simulink model "mass"  (R2025b)
settings: Solver=VariableStepAuto  StartTime=0.0  StopTime=10.0  RelTol=1e-3
PostLoadFcn:
  | rigid_body = importrobot('urdf\mass\urdf\mass.urdf');
  | rigid_body.DataFormat = 'column';
  | rigid_body.Gravity = [0 -9.81 0];
  | robot = get_robot_chain(rigid_body, 'mass','base_link');
  | robot.gravity = [0 -9.81 0];
libraries: aerolibanimutils x1
settings Model: Creator=Junch  LastModifiedBy=Junch

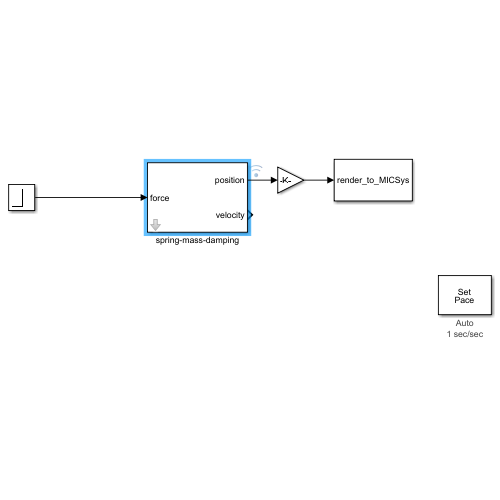
[thumbnail: Simulink's stored preview of the top-level diagram]
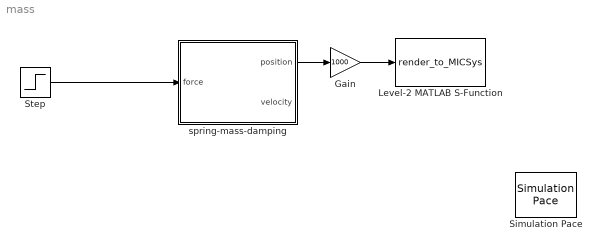
== system mass ==
  Gain : Gain  Gain=1000
  Level-2 MATLAB S-Function : M-S-Function  FunctionName=render_to_MICSys
  Simulation Pace : aerolibanimutils/Simulation Pace  SimulationPace=1  SleepMode=Auto  OutputPaceError=off  SampleTime=1/30
  Step : Step  SampleTime=0
  spring-mass-damping : Subsystem  mask{robot=robot, x0=0, Kd=1, Kp=5}
      mask prompts: x0 "intial position"; Kd "Kd (damping)"; Kp "Kp (spring)"
      mask DialogControl ParameterGroupVar Prompt: 参数
      mask Display:
      | port_label('output', 1, 'position');
      | port_label('output', 2, 'velocity');
      | port_label('input', 1, 'force');
  wires:
  Step/1 -> spring-mass-damping/1(force)
  spring-mass-damping/1(position) -> Gain/1
  Gain/1 -> Level-2 MATLAB S-Function/1

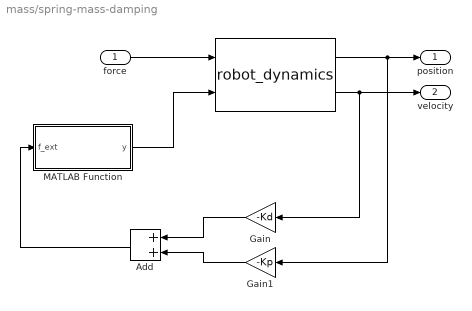
== system mass/spring-mass-damping ==
  force : Inport
  " " : M-S-Function  FunctionName=robot_dynamics  Parameters=robot, init_pos, init_vel  mask{robot=robot, init_pos=x0, init_vel=0}
      mask prompts: robot "robot struct:"; init_pos "init pos:"; init_vel "init velocity:"
      mask DialogControl ParameterGroupVar Prompt: 参数
      mask Display:
      | port_label('input', 1, 'control torque')
      | port_label('input', 2, 'external force')
      | port_label('output', 1, 'q')
      | port_label('output', 2, 'qd')
      | disp('Robot Dynamics');
  Add : Sum
  Gain : Gain  Gain=-Kd
  Gain1 : Gain  Gain=-Kp
  MATLAB Function : MATLAB Function  TreatAsAtomicUnit=on
  position : Outport
  velocity : Outport  Port=2
  wires:
  force/1 -> " "/1
  Gain/1 -> Add/1
  " "/2 -> velocity/1, Gain/1
  " "/1 -> Gain1/1, position/1
  Gain1/1 -> Add/2
  Add/1 -> MATLAB Function/1(f_ext)
  MATLAB Function/1(y) -> " "/2

== matlab function mass/spring-mass-damping/MATLAB Function ==
  data: f_ext input; y output
function y = fcn(f_ext)
y = [0, 0, 0, f_ext, 0, 0]';
